simulink model "project"  (R2022a)
settings: Solver=VariableStepAuto  StartTime=0.0  StopTime=60.0  RelTol=1e-3
model workspace (MAT data in the model file):
  A = [0  0.3  0.4  0.3; 0.3  0  0.5  0; 0.4  0.5  0  0.3; 0.3  0  0.3  0]
  b = [0.3; 0.2; 0.5; 0.4]
  c = [9; 7; 11; 7]
  diff = [1; 1; 1; 1]
  get = [17; 16; 16; 17]
  off = [20; 20; 20; 20]
  on = [19; 19; 19; 19]
  u = 6
settings Model: Creator=Hunter  LastModifiedBy=Hunter

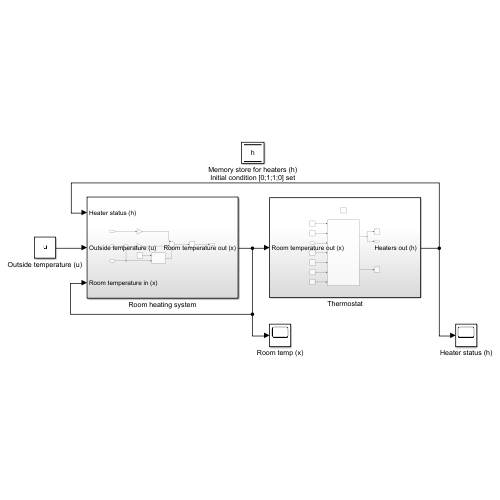
[thumbnail: Simulink's stored preview of the top-level diagram]
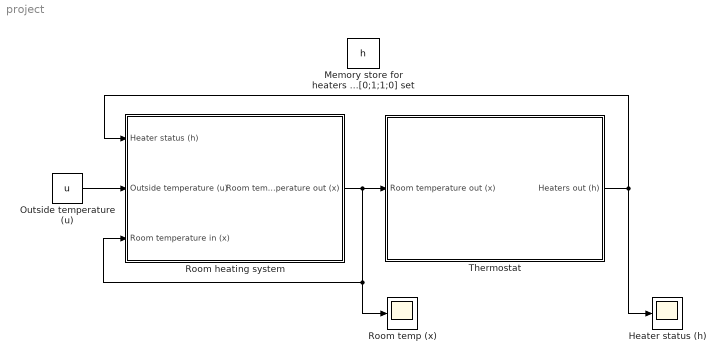
== system project ==
  Heater status (h) : Scope
  Memory store for heaters (h) Initial condition [0;1;1;0] set : DataStoreMemory  DataStoreName=h  WriteAfterWriteMsg=warning  InitialValue=[0;1;1;0]  ShowAdditionalParam=off
  Outside temperature (u) : Constant  Value=u
  Room heating system : Subsystem
  Room temp (x) : Scope
  Thermostat : Subsystem
  wires:
  Outside temperature (u)/1 -> Room heating system/2(Outside temperature (u))
  Room heating system/1(Room temperature out (x)) -> Thermostat/1(Room temperature out (x)), Room temp (x)/1, Room heating system/3(Room temperature in (x))
  Thermostat/1("Heaters out (h) ") -> Room heating system/1(Heater status (h)), Heater status (h)/1

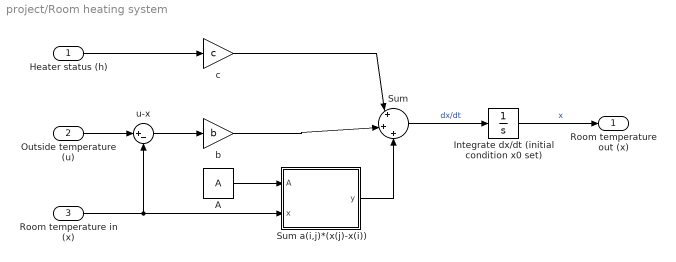
== system project/Room heating system ==
  Heater status (h) : Inport
  Outside temperature (u) : Inport  Port=2
  Room temperature in (x) : Inport  Port=3
  A : Constant  Value=A
  Integrate dx/dt (initial condition x0 set) : Integrator  InitialCondition=[16.5;16.5;16.5;16.5]
  Sum : Sum  Inputs=|+|+|+
  Sum a(i,j)*(x(j)-x(i)) : MATLAB Function  TreatAsAtomicUnit=on
  b : Gain  Gain=b
  c : Gain  Gain=c
  u-x : Sum  Inputs=|+-
  Room temperature out (x) : Outport
  wires:
  Heater status (h)/1 -> c/1
  c/1 -> Sum/1
  Outside temperature (u)/1 -> u-x/1
  Room temperature in (x)/1 -> u-x/2, Sum a(i,j)*(x(j)-x(i))/2(x)
  u-x/1 -> b/1
  b/1 -> Sum/2
  A/1 -> Sum a(i,j)*(x(j)-x(i))/1(A)
  Sum a(i,j)*(x(j)-x(i))/1(y) -> Sum/3
  Integrate dx/dt (initial condition x0 set)/1 -> Room temperature out (x)/1  "x"
  Sum/1 -> Integrate dx/dt (initial condition x0 set)/1  "dx/dt"

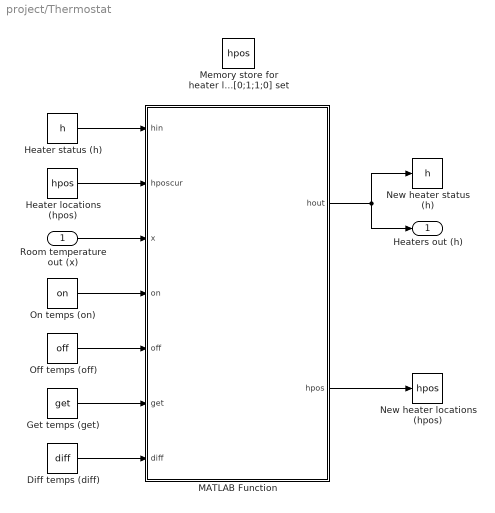
== system project/Thermostat ==
  Room temperature out (x) : Inport
  Diff temps (diff) : Constant  Value=diff
  Get temps (get) : Constant  Value=get
  Heater locations (hpos) : DataStoreRead  DataStoreName=hpos  IndexOptions=Index vector (dialog)  Indices=1  OutputSizes=1
  Heater status (h) : DataStoreRead  DataStoreName=h  IndexOptions=Index vector (dialog)  Indices=1  OutputSizes=1
  MATLAB Function : MATLAB Function  TreatAsAtomicUnit=on
  Memory store for heater locations (hpos) Initial condition [0;1;1;0] set : DataStoreMemory  DataStoreName=hpos  WriteAfterWriteMsg=warning  InitialValue=[0;1;1;0]  ShowAdditionalParam=off
  New heater locations (hpos) : DataStoreWrite  DataStoreName=hpos  IndexOptions=Index vector (dialog)  Indices=1  OutputSizes=1
  New heater status (h) : DataStoreWrite  DataStoreName=h  IndexOptions=Index vector (dialog)  Indices=1  OutputSizes=1
  Off temps (off) : Constant  Value=off
  On temps (on) : Constant  Value=on
  "Heaters out (h) " : Outport
  wires:
  Room temperature out (x)/1 -> MATLAB Function/3(x)
  Heater status (h)/1 -> MATLAB Function/1(hin)
  MATLAB Function/1(hout) -> New heater status (h)/1, "Heaters out (h) "/1
  On temps (on)/1 -> MATLAB Function/4(on)
  Off temps (off)/1 -> MATLAB Function/5(off)
  Get temps (get)/1 -> MATLAB Function/6(get)
  Diff temps (diff)/1 -> MATLAB Function/7(diff)
  MATLAB Function/2(hpos) -> New heater locations (hpos)/1
  Heater locations (hpos)/1 -> MATLAB Function/2(hposcur)

== matlab function project/Thermostat/MATLAB Function ==
  data: hin input; hposcur input; hout output; x input; on input; off input; get input; diff input; hpos output
function [hout, hpos] = fcn(hin, hposcur, x, on, off, get, diff)
hcur = hin;
hpos = hposcur;

for i = 1:4
    if (x(i) > off(i)) && (hin(i) == 1)
        hcur(i) = 0;
    end
    if (x(i) < on(i)) && (hposcur(i) == 1)
        hcur(i) = 1;
    end
end

for i = 1:4 
    for j = 1:4
        if i ~= j
            if (hposcur(i) == 0) && (hposcur(j) == 1) && (x(i) <= get(i)) && ((x(j) - x(i)) >= diff(i))
                hcur(j) = 0;
                hcur(i) = 1;
                hpos(j) = 0;
                hpos(i) = 1;
            end
        end
    end
end

hout = hcur;
end

== matlab function project/Room heating system/Sum a(i,j)*(x(j)-x(i)) ==
  data: A input; y output; x input
function y = fcn(A, x)
y = [0;0;0;0];
for i = 1:4 
    for j = 1:4
        if i ~= j
            y(i) = y(i) + A(i, j)*(x(j) - x(i));
        end
    end
end
end
